simulink model "das3implicit_test"  (Simulink 7.4)
settings: Solver=FixedStepDiscrete  StartTime=0.0  StopTime=4  FixedStep=0.001  RelTol=1e-3
libraries: simulink x2
settings Model: Creator=Dimitra  LastModifiedBy=Dimitra
settings DataIOCC: SaveOutput=off  SignalLogging=off  SaveTime=off

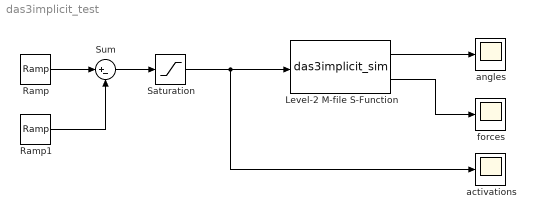
== system das3implicit_test ==
  Level-2 M-file S-Function : M-S-Function  FunctionName=das3implicit_sim
  Ramp : simulink/Sources/Ramp  SystemSampleTime=-1  slope=5  start=0  X0=zeros(138,1)
  Ramp1 : simulink/Sources/Ramp  SystemSampleTime=-1  slope=10000  start=2  X0=zeros(138,1)
  Saturation : Saturate  UpperLimit=1  LowerLimit=0
  Sum : Sum  Inputs=|+-  OutDataType=fixdt(1, 16)  OutScaling=2^0
  activations : Scope
      settings: SaveName=ScopeData2
  angles : Scope
      settings: YMin=-0.5  YMax=2  SaveName=angles  DataFormat=Array
  forces : Scope
      settings: YMin=-250  YMax=2000  SaveName=forces  DataFormat=Array
  wires:
  Ramp/1 -> Sum/1
  Ramp1/1 -> Sum/2
  Level-2 M-file S-Function/1 -> angles/1
  Level-2 M-file S-Function/2 -> forces/1
  Saturation/1 -> activations/1, Level-2 M-file S-Function/1
  Sum/1 -> Saturation/1
